simulink library "nort_sysgenlib"  (Simulink 6.5)
undefined symbols (not defined in the file or in its folder): Down, Up
libraries: xbsIndex_r4 x338, nort_sysgenlib x10
(part 2 of 2)

== system nort_sysgenlib/UnConcat32 ==
  note: Unconcat32: March 7, 2008
  In32 : Inport
  Convert : xbsIndex_r4/Convert  arith_type="Signed  (2's comp)"  n_bits=32  bin_pt=0  quantization=Truncate  overflow=Wrap  latency=0  dbl_ovrd=off  pipeline=off  block_type=convert
      settings: block_version=9.2.01
  Convert1 : xbsIndex_r4/Convert  arith_type="Signed  (2's comp)"  n_bits=32  bin_pt=0  quantization=Truncate  overflow=Wrap  latency=0  dbl_ovrd=off  pipeline=off  block_type=convert
      settings: block_version=9.2.01
  Convert2 : xbsIndex_r4/Convert  arith_type="Signed  (2's comp)"  n_bits=32  bin_pt=0  quantization=Truncate  overflow=Wrap  latency=0  dbl_ovrd=off  pipeline=off  block_type=convert
      settings: block_version=9.2.01
  Slice3 : xbsIndex_r4/Slice  nbits=32  boolean_output=off  mode=Lower Bit Location + Width  bit1=0  base1=MSB of Input  bit0=64  base0=LSB of Input  dbl_ovrd=off  block_type=slice
      settings: infoedit="Extracts a given range of bits from each input sample and presents it at the output.  The output type is ordinarily unsigned with binary point at zero, but can be Boolean when the slice is one bit wide.<P><P>Hardware notes: In hardware this block costs nothing."  block_version=9.2.01
  Slice4 : xbsIndex_r4/Slice  nbits=32  boolean_output=off  mode=Lower Bit Location + Width  bit1=0  base1=MSB of Input  bit0=32  base0=LSB of Input  dbl_ovrd=off  block_type=slice
      settings: infoedit="Extracts a given range of bits from each input sample and presents it at the output.  The output type is ordinarily unsigned with binary point at zero, but can be Boolean when the slice is one bit wide.<P><P>Hardware notes: In hardware this block costs nothing."  block_version=9.2.01
  Slice5 : xbsIndex_r4/Slice  nbits=32  boolean_output=off  mode=Lower Bit Location + Width  bit1=0  base1=MSB of Input  bit0=0  base0=LSB of Input  dbl_ovrd=off  block_type=slice
      settings: infoedit="Extracts a given range of bits from each input sample and presents it at the output.  The output type is ordinarily unsigned with binary point at zero, but can be Boolean when the slice is one bit wide.<P><P>Hardware notes: In hardware this block costs nothing."  block_version=9.2.01
  Out0 : Outport
  Out1 : Outport  Port=2
  Out2 : Outport  Port=3
  wires:
  Convert2/1 -> Out2/1
  Convert1/1 -> Out1/1
  Convert/1 -> Out0/1
  Slice5/1 -> Convert2/1
  Slice4/1 -> Convert1/1
  Slice3/1 -> Convert/1
  In32/1 -> Slice5/1, Slice4/1, Slice3/1

== system nort_sysgenlib/arp_ssp ==
  LVDS : Inport
  Signal : Outport
  ADOOR : Outport  Port=2
  wires:
  LVDS/1 -> Signal/1

== system nort_sysgenlib/ssp_ad_preaddr ==
  Signal : Inport
  ADOOR : Inport  Port=2
  TrigLevel : Inport  Port=3
  NAvg : Inport  Port=4
  RE : Inport  Port=5
  Reset : Inport  Port=6
  Trigger : Inport  Port=7
  PA_Out : Outport
  LvlGreater : Outport  Port=2
  wires:
  Signal/1 -> PA_Out/1

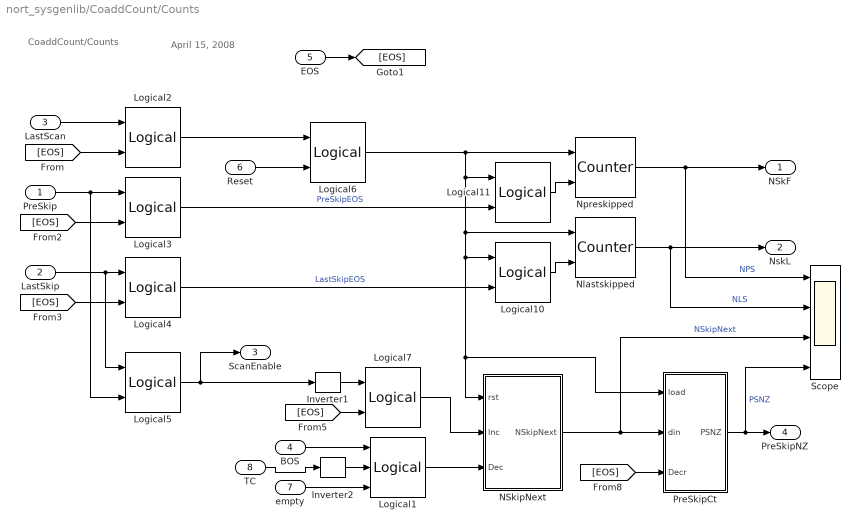
== system nort_sysgenlib/CoaddCount/Counts ==
  note: April 15, 2008
  note: CoaddCount/Counts
  PreSkip : Inport
  LastSkip : Inport  Port=2
  LastScan : Inport  Port=3
  BOS : Inport  Port=4
  EOS : Inport  Port=5
  Reset : Inport  Port=6
  empty : Inport  Port=7
  TC : Inport  Port=8
  Inverter1 : xbsIndex_r4/Inverter  en=off  latency=0  dbl_ovrd=off  block_type=inv
      settings: block_version=9.2.01
  Inverter2 : xbsIndex_r4/Inverter  en=off  latency=0  dbl_ovrd=off  block_type=inv
      settings: block_version=9.2.01
  Logical1 : xbsIndex_r4/Logical  logical_function=AND  inputs=3  en=off  latency=0  precision=Full  arith_type=Unsigned  n_bits=16  bin_pt=0  align_bp=on  dbl_ovrd=off  block_type=logical
      settings: block_version=9.2.01
  Logical10 : xbsIndex_r4/Logical  logical_function=OR  inputs=2  en=off  latency=0  precision=Full  arith_type=Unsigned  n_bits=16  bin_pt=0  align_bp=on  dbl_ovrd=off  block_type=logical
      settings: block_version=9.2.01
  Logical11 : xbsIndex_r4/Logical  logical_function=OR  inputs=2  en=off  latency=0  precision=Full  arith_type=Unsigned  n_bits=16  bin_pt=0  align_bp=on  dbl_ovrd=off  block_type=logical
      settings: block_version=9.2.01
  Logical{2..4,7} (4 alike) : xbsIndex_r4/Logical  logical_function=AND  inputs=2  en=off  latency=0  precision=Full  arith_type=Unsigned  n_bits=16  bin_pt=0  align_bp=on  dbl_ovrd=off  block_type=logical
      settings: block_version=9.2.01
  Logical5 : xbsIndex_r4/Logical  logical_function=NOR  inputs=2  en=off  latency=0  precision=Full  arith_type=Unsigned  n_bits=16  bin_pt=0  align_bp=on  dbl_ovrd=off  block_type=logical
      settings: block_version=9.2.01
  Logical6 : xbsIndex_r4/Logical  logical_function=OR  inputs=2  en=off  latency=0  precision=Full  arith_type=Unsigned  n_bits=16  bin_pt=0  align_bp=on  dbl_ovrd=off  block_type=logical
      settings: block_version=9.2.01
  NSkipNext : Subsystem
  Nlastskipped : xbsIndex_r4/Counter  cnt_type=Free Running  cnt_to=Inf  operation=Up  start_count=0  cnt_by_val=1  arith_type=Unsigned  n_bits=16  bin_pt=0  load_pin=off  rst=on  en=on  explicit_period=on  period=1  dbl_ovrd=off  use_behavioral_HDL=off  use_rpm=off  block_type=counter
      settings: block_version=9.2.01
  Npreskipped : xbsIndex_r4/Counter  cnt_type=Free Running  cnt_to=Inf  operation=Up  start_count=0  cnt_by_val=1  arith_type=Unsigned  n_bits=16  bin_pt=0  load_pin=off  rst=on  en=on  explicit_period=on  period=1  dbl_ovrd=off  use_behavioral_HDL=off  use_rpm=off  block_type=counter
      settings: block_version=9.2.01
  PreSkipCt : Subsystem
  Scope : Scope  NumInputPorts=4
      settings: TimeRange=5000  YMin=-0.25~-5~0~-5  YMax=1.25~5~15~5
  NSkF : Outport
  NskL : Outport  Port=2
  ScanEnable : Outport  Port=3
  PreSkipNZ : Outport  Port=4
  wires:
  Logical1/1 -> NSkipNext/3(Dec)
  empty/1 -> Logical1/3
  TC/1 -> Inverter2/1
  Inverter2/1 -> Logical1/2
  BOS/1 -> Logical1/1
  Logical7/1 -> NSkipNext/2(Inc)
  [EOS] -> Logical7/2
  Inverter1/1 -> Logical7/1
  [EOS] -> PreSkipCt/3(Decr)
  Reset/1 -> Logical6/2
  [EOS] -> Logical4/2
  [EOS] -> Logical3/2
  LastScan/1 -> Logical2/1
  [EOS] -> Logical2/2
  Logical6/1 -> Npreskipped/1, Nlastskipped/1, NSkipNext/1(rst), PreSkipCt/1(load), Logical10/1, Logical11/1
  Logical2/1 -> Logical6/1
  LastSkip/1 -> Logical5/1, Logical4/1
  Logical4/1 -> Logical10/2  "LastSkipEOS"
  Logical3/1 -> Logical11/2  "PreSkipEOS"
  PreSkip/1 -> Logical5/2, Logical3/1
  Logical5/1 -> Inverter1/1, ScanEnable/1
  PreSkipCt/1(PSNZ) -> Scope/4, PreSkipNZ/1  "PSNZ"
  EOS/1 -> [EOS]
  NSkipNext/1(NSkipNext) -> Scope/3, PreSkipCt/2(din)  "NSkipNext"
  Nlastskipped/1 -> Scope/2, NskL/1  "NLS"
  Npreskipped/1 -> Scope/1, NSkF/1  "NPS"
  Logical10/1 -> Nlastskipped/2
  Logical11/1 -> Npreskipped/2

== system nort_sysgenlib/CoaddCount/ScanCount ==
  note: March 6, 2008
  note: CoaddCount/ScanCount
  rst : Inport
  NC : Inport  Port=2
  en : Inport  Port=3
  Ncoadding : xbsIndex_r4/Counter  cnt_type=Free Running  cnt_to=Inf  operation=Up  start_count=1  cnt_by_val=1  arith_type=Unsigned  n_bits=14  bin_pt=0  load_pin=off  rst=on  en=on  explicit_period=on  period=1  dbl_ovrd=off  use_behavioral_HDL=off  use_rpm=off  block_type=counter
      settings: block_version=9.2.01
  Relational : xbsIndex_r4/Relational  mode=a=b  en=off  latency=0  dbl_ovrd=off  block_type=relational
      settings: block_version=9.2.01
  TC : Outport
  wires:
  en/1 -> Ncoadding/2
  Relational/1 -> TC/1
  rst/1 -> Ncoadding/1
  Ncoadding/1 -> Relational/2
  NC/1 -> Relational/1

== system nort_sysgenlib/PreAdder/Count ==
  note: February 27, 2008
  note: ssp_ad_preaddr/State
      | Simplified 2/27
      | EOSum is true on TC only
  NA : Inport
  Reset : Inport  Port=2
  Constant : xbsIndex_r4/Constant  arith_type=Unsigned  const=0  n_bits=7  bin_pt=0  explicit_period=off  period=1  equ=P=C  opselect=C  inp2=PCIN>>17  opr=+  inp1=P  carry=CIN  dbl_ovrd=off  block_type=constant
      settings: block_version=9.1.01
  Counter : xbsIndex_r4/Counter  cnt_type=Free Running  cnt_to=Inf  operation=Down  start_count=0  cnt_by_val=1  arith_type=Unsigned  n_bits=8  bin_pt=0  load_pin=on  rst=off  en=off  explicit_period=on  period=1  dbl_ovrd=off  use_behavioral_HDL=off  use_rpm=off  block_type=counter
      settings: block_version=9.1.01
  Inverter : xbsIndex_r4/Inverter  en=off  latency=0  dbl_ovrd=off  block_type=inv
      settings: block_version=9.2.01
  Logical : xbsIndex_r4/Logical  logical_function=OR  inputs=2  en=off  latency=0  precision=Full  arith_type=Unsigned  n_bits=16  bin_pt=0  align_bp=on  dbl_ovrd=off  block_type=logical
      settings: block_version=9.2.01
  Logical1 : xbsIndex_r4/Logical  logical_function=AND  inputs=2  en=off  latency=0  precision=Full  arith_type=Unsigned  n_bits=16  bin_pt=0  align_bp=on  dbl_ovrd=off  block_type=logical
      settings: block_version=9.2.01
  Relational : xbsIndex_r4/Relational  mode=a=b  en=off  latency=0  dbl_ovrd=off  block_type=relational
      settings: block_version=9.1.01
  NewData : Outport
  wires:
  Inverter/1 -> Logical1/2
  Logical1/1 -> NewData/1
  Logical/1 -> Counter/1
  Reset/1 -> Inverter/1, Logical/2  "Reset"
  NA/1 -> Counter/2
  Relational/1 -> Logical1/1, Logical/1  "TC"
  Constant/1 -> Relational/2
  Counter/1 -> Relational/1

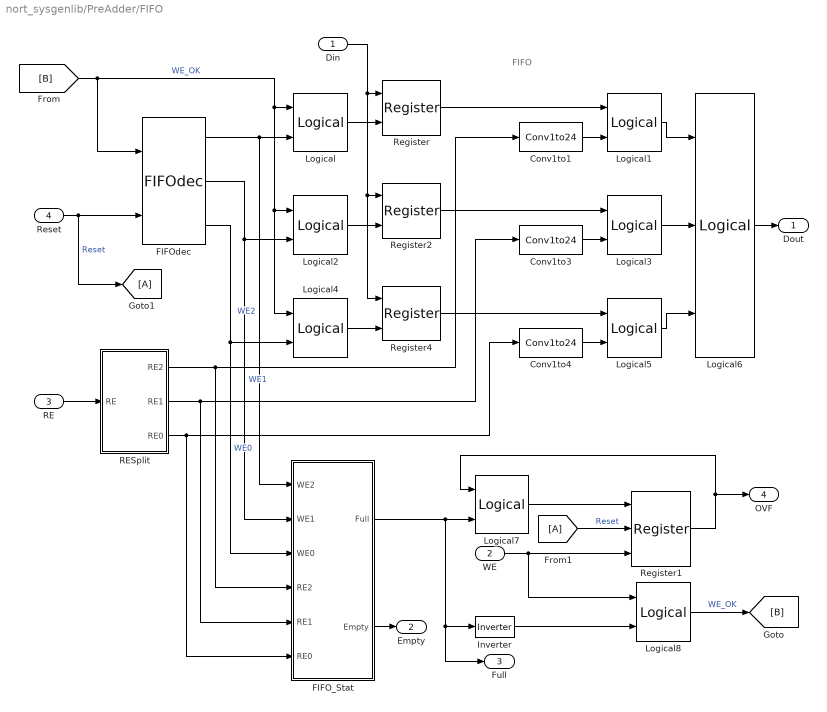
== system nort_sysgenlib/PreAdder/FIFO ==
  note: FIFO
  Din : Inport
  WE : Inport  Port=2
  RE : Inport  Port=3
  Reset : Inport  Port=4
  Conv1to1 : nort_sysgenlib/Conv1to24  SystemSampleTime=-1
  Conv1to3 : nort_sysgenlib/Conv1to24  SystemSampleTime=-1
  Conv1to4 : nort_sysgenlib/Conv1to24  SystemSampleTime=-1
  FIFO_Stat : Subsystem
  FIFOdec : nort_sysgenlib/FIFOdec  SystemSampleTime=-1
  Inverter : xbsIndex_r4/Inverter  en=off  latency=0  dbl_ovrd=off  block_type=inv
      settings: block_version=9.2.01
  Logical{,1..5,8} (7 alike) : xbsIndex_r4/Logical  logical_function=AND  inputs=2  en=off  latency=0  precision=Full  arith_type=Unsigned  n_bits=16  bin_pt=0  align_bp=on  dbl_ovrd=off  block_type=logical
      settings: block_version=9.2.01
  Logical6 : xbsIndex_r4/Logical  logical_function=OR  inputs=3  en=off  latency=0  precision=Full  arith_type=Unsigned  n_bits=16  bin_pt=0  align_bp=on  dbl_ovrd=off  block_type=logical
      settings: block_version=9.2.01
  Logical7 : xbsIndex_r4/Logical  logical_function=OR  inputs=2  en=off  latency=0  precision=Full  arith_type=Unsigned  n_bits=16  bin_pt=0  align_bp=on  dbl_ovrd=off  block_type=logical
      settings: block_version=9.2.01
  RESplit : Subsystem
  Register : xbsIndex_r4/Register  init=0  rst=off  en=on  dbl_ovrd=off  block_type=register
      settings: block_version=9.2.01
  Register1 : xbsIndex_r4/Register  init=0  rst=on  en=on  dbl_ovrd=off  block_type=register
      settings: block_version=9.2.01
  Register2 : xbsIndex_r4/Register  init=0  rst=off  en=on  dbl_ovrd=off  block_type=register
      settings: block_version=9.2.01
  Register4 : xbsIndex_r4/Register  init=0  rst=off  en=on  dbl_ovrd=off  block_type=register
      settings: block_version=9.2.01
  Dout : Outport
  Empty : Outport  Port=2
  Full : Outport  Port=3
  OVF : Outport  Port=4
  wires:
  [B] -> FIFOdec/1, Logical2/1, Logical4/1, Logical/1  "WE_OK"
  Logical8/1 -> [B]  "WE_OK"
  [A] -> Register1/2  "Reset"
  Inverter/1 -> Logical8/2
  FIFO_Stat/1(Full) -> Full/1, Inverter/1, Logical7/2
  FIFO_Stat/2(Empty) -> Empty/1
  Logical7/1 -> Register1/1
  WE/1 -> Logical8/1, Register1/3
  Register1/1 -> Logical7/1, OVF/1
  RE/1 -> RESplit/1(RE)
  Reset/1 -> FIFOdec/2, [A]  "Reset"
  Logical6/1 -> Dout/1
  Logical5/1 -> Logical6/3
  Logical3/1 -> Logical6/2
  Logical1/1 -> Logical6/1
  RESplit/1(RE2) -> FIFO_Stat/4(RE2), Conv1to1/1
  Register4/1 -> Logical5/1
  Register2/1 -> Logical3/1
  Conv1to4/1 -> Logical5/2
  FIFOdec/3 -> FIFO_Stat/3(WE0), Logical4/2  "WE0"
  Logical4/1 -> Register4/2
  Conv1to3/1 -> Logical3/2
  FIFOdec/2 -> FIFO_Stat/2(WE1), Logical2/2  "WE1"
  Logical2/1 -> Register2/2
  Register/1 -> Logical1/1
  Conv1to1/1 -> Logical1/2
  RESplit/3(RE0) -> FIFO_Stat/6(RE0), Conv1to4/1
  RESplit/2(RE1) -> FIFO_Stat/5(RE1), Conv1to3/1
  FIFOdec/1 -> FIFO_Stat/1(WE2), Logical/2  "WE2"
  Din/1 -> Register4/1, Register2/1, Register/1
  Logical/1 -> Register/2

== system nort_sysgenlib/PreAdder/State ==
  note: February 27, 2008
  note: PreAdder State
  ResIn : Inport
  Trigger : Inport  Port=2
  ActiveSt : xbsIndex_r4/Register  init=0  rst=off  en=off  dbl_ovrd=off  block_type=register
      settings: block_version=9.2.01
  Armed : xbsIndex_r4/Register  init=0  rst=off  en=off  dbl_ovrd=off  block_type=register
      settings: block_version=9.2.01
  Inverter1 : xbsIndex_r4/Inverter  en=off  latency=0  dbl_ovrd=off  block_type=inv
      settings: block_version=9.2.01
  Inverter2 : xbsIndex_r4/Inverter  en=off  latency=0  dbl_ovrd=off  block_type=inv
      settings: block_version=9.2.01
  Inverter3 : xbsIndex_r4/Inverter  en=off  latency=0  dbl_ovrd=off  block_type=inv
      settings: block_version=9.2.01
  Logical{1,4,6..7} (4 alike) : xbsIndex_r4/Logical  logical_function=AND  inputs=2  en=off  latency=0  precision=Full  arith_type=Unsigned  n_bits=16  bin_pt=0  align_bp=on  dbl_ovrd=off  block_type=logical
      settings: block_version=9.2.01
  Logical5 : xbsIndex_r4/Logical  logical_function=OR  inputs=2  en=off  latency=0  precision=Full  arith_type=Unsigned  n_bits=16  bin_pt=0  align_bp=on  dbl_ovrd=off  block_type=logical
      settings: block_version=9.2.01
  Logical8 : xbsIndex_r4/Logical  logical_function=OR  inputs=2  en=off  latency=0  precision=Full  arith_type=Unsigned  n_bits=16  bin_pt=0  align_bp=on  dbl_ovrd=off  block_type=logical
      settings: block_version=9.2.01
  ResetSt : xbsIndex_r4/Register  init=0  rst=off  en=off  dbl_ovrd=off  block_type=register
      settings: block_version=9.2.01
  Inactive : Outport
  Reset : Outport  Port=2
  wires:
  Inverter2/1 -> Inactive/1
  Logical1/1 -> Logical8/1
  Inverter3/1 -> Logical6/1
  Logical8/1 -> Logical7/2
  Logical7/1 -> Inverter2/1, ActiveSt/1
  ActiveSt/1 -> Logical8/2
  Armed/1 -> Logical1/1, Logical6/2
  Logical6/1 -> Logical5/2
  Logical5/1 -> Logical4/1
  Inverter1/1 -> Logical4/2, Logical7/1
  Logical4/1 -> Armed/1
  ResIn/1 -> ResetSt/1, Inverter1/1  "Reset_In"
  Trigger/1 -> Logical1/2, Inverter3/1  "Trigger"
  ResetSt/1 -> Logical5/1, Reset/1

== system nort_sysgenlib/PreAdderA/Count ==
  note: April 16, 2008
  note: ssp_ad_preaddr/State
      | Simplified 2/27
      | EOSum is true on TC only
  Reset : Inport
  NA : Inport  Port=2
  Constant : xbsIndex_r4/Constant  arith_type=Unsigned  const=0  n_bits=7  bin_pt=0  explicit_period=off  period=1  equ=P=C  opselect=C  inp2=PCIN>>17  opr=+  inp1=P  carry=CIN  dbl_ovrd=off  block_type=constant
      settings: block_version=9.1.01
  Counter : xbsIndex_r4/Counter  cnt_type=Free Running  cnt_to=Inf  operation=Down  start_count=0  cnt_by_val=1  arith_type=Unsigned  n_bits=8  bin_pt=0  load_pin=on  rst=off  en=off  explicit_period=on  period=1  dbl_ovrd=off  use_behavioral_HDL=off  use_rpm=off  block_type=counter
      settings: block_version=9.1.01
  Inverter : xbsIndex_r4/Inverter  en=off  latency=0  dbl_ovrd=off  block_type=inv
      settings: block_version=9.2.01
  Logical : xbsIndex_r4/Logical  logical_function=OR  inputs=2  en=off  latency=0  precision=Full  arith_type=Unsigned  n_bits=16  bin_pt=0  align_bp=on  dbl_ovrd=off  block_type=logical
      settings: block_version=9.2.01
  Logical1 : xbsIndex_r4/Logical  logical_function=AND  inputs=2  en=off  latency=0  precision=Full  arith_type=Unsigned  n_bits=16  bin_pt=0  align_bp=on  dbl_ovrd=off  block_type=logical
      settings: block_version=9.2.01
  Relational : xbsIndex_r4/Relational  mode=a=b  en=off  latency=0  dbl_ovrd=off  block_type=relational
      settings: block_version=9.1.01
  NewData : Outport
  wires:
  Inverter/1 -> Logical1/2
  Logical1/1 -> NewData/1
  Logical/1 -> Counter/1
  Reset/1 -> Inverter/1, Logical/2  "Reset"
  NA/1 -> Counter/2
  Relational/1 -> Logical1/1, Logical/1  "TC"
  Constant/1 -> Relational/2
  Counter/1 -> Relational/1

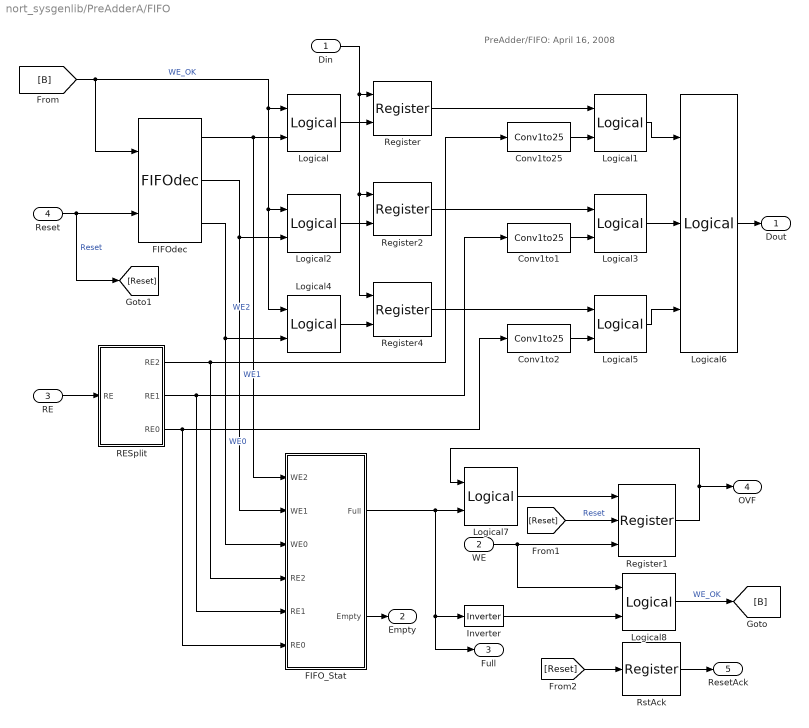
== system nort_sysgenlib/PreAdderA/FIFO ==
  note: PreAdder/FIFO: April 16, 2008
  Din : Inport
  WE : Inport  Port=2
  RE : Inport  Port=3
  Reset : Inport  Port=4
  Conv1to1 : nort_sysgenlib/Conv1to25  SystemSampleTime=-1
  Conv1to2 : nort_sysgenlib/Conv1to25  SystemSampleTime=-1
  Conv1to25 : nort_sysgenlib/Conv1to25  SystemSampleTime=-1
  FIFO_Stat : Subsystem
  FIFOdec : nort_sysgenlib/FIFOdec  SystemSampleTime=-1
  Inverter : xbsIndex_r4/Inverter  en=off  latency=0  dbl_ovrd=off  block_type=inv
      settings: block_version=9.2.01
  Logical{,1..5,8} (7 alike) : xbsIndex_r4/Logical  logical_function=AND  inputs=2  en=off  latency=0  precision=Full  arith_type=Unsigned  n_bits=16  bin_pt=0  align_bp=on  dbl_ovrd=off  block_type=logical
      settings: block_version=9.2.01
  Logical6 : xbsIndex_r4/Logical  logical_function=OR  inputs=3  en=off  latency=0  precision=Full  arith_type=Unsigned  n_bits=16  bin_pt=0  align_bp=on  dbl_ovrd=off  block_type=logical
      settings: block_version=9.2.01
  Logical7 : xbsIndex_r4/Logical  logical_function=OR  inputs=2  en=off  latency=0  precision=Full  arith_type=Unsigned  n_bits=16  bin_pt=0  align_bp=on  dbl_ovrd=off  block_type=logical
      settings: block_version=9.2.01
  RESplit : Subsystem
  Register : xbsIndex_r4/Register  init=0  rst=off  en=on  dbl_ovrd=off  block_type=register
      settings: block_version=9.2.01
  Register1 : xbsIndex_r4/Register  init=0  rst=on  en=on  dbl_ovrd=off  block_type=register
      settings: block_version=9.2.01
  Register2 : xbsIndex_r4/Register  init=0  rst=off  en=on  dbl_ovrd=off  block_type=register
      settings: block_version=9.2.01
  Register4 : xbsIndex_r4/Register  init=0  rst=off  en=on  dbl_ovrd=off  block_type=register
      settings: block_version=9.2.01
  RstAck : xbsIndex_r4/Register  init=0  rst=off  en=off  dbl_ovrd=off  block_type=register
      settings: block_version=9.2.01
  Dout : Outport
  Empty : Outport  Port=2
  Full : Outport  Port=3
  OVF : Outport  Port=4
  ResetAck : Outport  Port=5
  wires:
  [Reset] -> RstAck/1
  RstAck/1 -> ResetAck/1
  [B] -> FIFOdec/1, Logical2/1, Logical4/1, Logical/1  "WE_OK"
  Logical8/1 -> [B]  "WE_OK"
  [Reset] -> Register1/2  "Reset"
  Inverter/1 -> Logical8/2
  FIFO_Stat/1(Full) -> Full/1, Inverter/1, Logical7/2
  FIFO_Stat/2(Empty) -> Empty/1
  Logical7/1 -> Register1/1
  WE/1 -> Logical8/1, Register1/3
  Register1/1 -> Logical7/1, OVF/1
  RE/1 -> RESplit/1(RE)
  Reset/1 -> FIFOdec/2, [Reset]  "Reset"
  Logical6/1 -> Dout/1
  Logical5/1 -> Logical6/3
  Logical3/1 -> Logical6/2
  Logical1/1 -> Logical6/1
  RESplit/1(RE2) -> FIFO_Stat/4(RE2), Conv1to25/1
  Register4/1 -> Logical5/1
  Register2/1 -> Logical3/1
  Conv1to2/1 -> Logical5/2
  FIFOdec/3 -> FIFO_Stat/3(WE0), Logical4/2  "WE0"
  Logical4/1 -> Register4/2
  Conv1to1/1 -> Logical3/2
  FIFOdec/2 -> FIFO_Stat/2(WE1), Logical2/2  "WE1"
  Logical2/1 -> Register2/2
  Register/1 -> Logical1/1
  Conv1to25/1 -> Logical1/2
  RESplit/3(RE0) -> FIFO_Stat/6(RE0), Conv1to2/1
  RESplit/2(RE1) -> FIFO_Stat/5(RE1), Conv1to1/1
  FIFOdec/1 -> FIFO_Stat/1(WE2), Logical/2  "WE2"
  Din/1 -> Register4/1, Register2/1, Register/1
  Logical/1 -> Register/2

== system nort_sysgenlib/PreAdderA/State ==
  note: April 16, 2008
  note: PreAdder State
  Trigger : Inport
  ResIn : Inport  Port=2
  ActiveSt : xbsIndex_r4/Register  init=0  rst=off  en=off  dbl_ovrd=off  block_type=register
      settings: block_version=9.2.01
  Armed : xbsIndex_r4/Register  init=0  rst=off  en=off  dbl_ovrd=off  block_type=register
      settings: block_version=9.2.01
  Inverter1 : xbsIndex_r4/Inverter  en=off  latency=0  dbl_ovrd=off  block_type=inv
      settings: block_version=9.2.01
  Inverter2 : xbsIndex_r4/Inverter  en=off  latency=0  dbl_ovrd=off  block_type=inv
      settings: block_version=9.2.01
  Inverter3 : xbsIndex_r4/Inverter  en=off  latency=0  dbl_ovrd=off  block_type=inv
      settings: block_version=9.2.01
  Logical{1,4,6..7} (4 alike) : xbsIndex_r4/Logical  logical_function=AND  inputs=2  en=off  latency=0  precision=Full  arith_type=Unsigned  n_bits=16  bin_pt=0  align_bp=on  dbl_ovrd=off  block_type=logical
      settings: block_version=9.2.01
  Logical5 : xbsIndex_r4/Logical  logical_function=OR  inputs=2  en=off  latency=0  precision=Full  arith_type=Unsigned  n_bits=16  bin_pt=0  align_bp=on  dbl_ovrd=off  block_type=logical
      settings: block_version=9.2.01
  Logical8 : xbsIndex_r4/Logical  logical_function=OR  inputs=2  en=off  latency=0  precision=Full  arith_type=Unsigned  n_bits=16  bin_pt=0  align_bp=on  dbl_ovrd=off  block_type=logical
      settings: block_version=9.2.01
  ResetSt : xbsIndex_r4/Register  init=0  rst=off  en=off  dbl_ovrd=off  block_type=register
      settings: block_version=9.2.01
  Inactive : Outport
  Reset : Outport  Port=2
  wires:
  Inverter2/1 -> Inactive/1
  Logical1/1 -> Logical8/1
  Inverter3/1 -> Logical6/1
  Logical8/1 -> Logical7/2
  Logical7/1 -> Inverter2/1, ActiveSt/1
  ActiveSt/1 -> Logical8/2
  Armed/1 -> Logical1/1, Logical6/2
  Logical6/1 -> Logical5/2
  Logical5/1 -> Logical4/1
  Inverter1/1 -> Logical4/2, Logical7/1
  Logical4/1 -> Armed/1
  ResIn/1 -> ResetSt/1, Inverter1/1  "Reset_In"
  Trigger/1 -> Logical1/2, Inverter3/1  "Trigger"
  ResetSt/1 -> Logical5/1, Reset/1

== system nort_sysgenlib/StateShifter/MuxAddrCalc ==
  note: MuxAddrCalc: March 7, 2008
  SHsel : Inport
  St0 : Inport  Port=2
  St1 : Inport  Port=3
  St2 : Inport  Port=4
  AddSub : xbsIndex_r4/AddSub  mode=Addition  use_carryin=off  use_carryout=off  en=off  latency=0  precision=Full  arith_type=Unsigned  n_bits=16  bin_pt=14  quantization=Truncate  overflow=Wrap  dbl_ovrd=off  use_behavioral_HDL=off  pipelined=off  use_rpm=on  block_type=addsub
      settings: block_version=9.2.01
  Concat : xbsIndex_r4/Concat  num_inputs=2  dbl_ovrd=off  block_type=concat
      settings: block_version=9.2.01
  Logical1 : xbsIndex_r4/Logical  logical_function=OR  inputs=2  en=off  latency=0  precision=Full  arith_type=Unsigned  n_bits=16  bin_pt=0  align_bp=on  dbl_ovrd=off  block_type=logical
      settings: block_version=9.2.01
  Logical2 : xbsIndex_r4/Logical  logical_function=OR  inputs=2  en=off  latency=0  precision=Full  arith_type=Unsigned  n_bits=16  bin_pt=0  align_bp=on  dbl_ovrd=off  block_type=logical
      settings: block_version=9.2.01
  MuxSel : Outport
  wires:
  St0/1 -> Logical1/1
  St1/1 -> Logical2/1
  AddSub/1 -> MuxSel/1
  SHsel/1 -> AddSub/1
  Concat/1 -> AddSub/2
  Logical1/1 -> Concat/2
  Logical2/1 -> Concat/1
  St2/1 -> Logical2/2, Logical1/2

== system nort_sysgenlib/StateShifter/ShiftHeader ==
  note: March 7, 2008
  note: ShiftHeader
  StI : Inport
  StSH : Inport  Port=2
  notfull : Inport  Port=3
  Constant : xbsIndex_r4/Constant  arith_type=Unsigned  const=5  n_bits=4  bin_pt=0  explicit_period=off  period=1  equ=P=C  opselect=C  inp2=PCIN>>17  opr=+  inp1=P  carry=CIN  dbl_ovrd=off  block_type=constant
      settings: block_version=9.2.01
  Counter : xbsIndex_r4/Counter  cnt_type=Free Running  cnt_to=Inf  operation=Up  start_count=0  cnt_by_val=1  arith_type=Unsigned  n_bits=3  bin_pt=0  load_pin=off  rst=on  en=on  explicit_period=on  period=1  dbl_ovrd=off  use_behavioral_HDL=off  use_rpm=off  block_type=counter
      settings: block_version=9.2.01
  Logical1 : xbsIndex_r4/Logical  logical_function=AND  inputs=2  en=off  latency=0  precision=Full  arith_type=Unsigned  n_bits=16  bin_pt=0  align_bp=on  dbl_ovrd=off  block_type=logical
      settings: block_version=9.2.01
  Logical2 : xbsIndex_r4/Logical  logical_function=AND  inputs=2  en=off  latency=0  precision=Full  arith_type=Unsigned  n_bits=16  bin_pt=0  align_bp=on  dbl_ovrd=off  block_type=logical
      settings: block_version=9.2.01
  Relational : xbsIndex_r4/Relational  mode=a=b  en=off  latency=0  dbl_ovrd=off  block_type=relational
      settings: block_version=9.2.01
  SHdone : Outport
  SHSel : Outport  Port=2
  wires:
  Logical2/1 -> SHdone/1
  Relational/1 -> Logical2/1
  Constant/1 -> Relational/2
  notfull/1 -> Logical2/2, Logical1/2
  StSH/1 -> Logical1/1
  StI/1 -> Counter/1
  Logical1/1 -> Counter/2
  Counter/1 -> SHSel/1, Relational/1

== system nort_sysgenlib/Triggering/AutoTrig ==
  note: AutoTrigger Circuit: May 28, 2008
  Trig : Inport
  AutoEn : Inport  Port=2
  Constant : xbsIndex_r4/Constant  arith_type=Unsigned  const=0  n_bits=9  bin_pt=0  explicit_period=off  period=1  equ=P=C  opselect=C  inp2=PCIN>>17  opr=+  inp1=P  carry=CIN  dbl_ovrd=off  block_type=constant
      settings: block_version=9.1.01
  Counter : xbsIndex_r4/Counter  cnt_type=Free Running  cnt_to=Inf  operation=Down  start_count=10000000  cnt_by_val=1  arith_type=Unsigned  n_bits=24  bin_pt=0  load_pin=off  rst=on  en=off  explicit_period=on  period=1  dbl_ovrd=off  use_behavioral_HDL=off  use_rpm=off  block_type=counter
      settings: block_version=9.1.01
  Delay : xbsIndex_r4/Delay  en=off  latency=1  dbl_ovrd=off  reg_retiming=off  block_type=delay
      settings: block_version=9.2.01
  Inverter : xbsIndex_r4/Inverter  en=off  latency=0  dbl_ovrd=off  block_type=inv
      settings: block_version=9.1.01
  Inverter1 : xbsIndex_r4/Inverter  en=off  latency=0  dbl_ovrd=off  block_type=inv
      settings: block_version=9.2.01
  Logical1 : xbsIndex_r4/Logical  logical_function=AND  inputs=2  en=off  latency=0  precision=Full  arith_type=Unsigned  n_bits=16  bin_pt=0  align_bp=on  dbl_ovrd=off  block_type=logical
      settings: block_version=9.1.01
  Logical2 : xbsIndex_r4/Logical  logical_function=OR  inputs=2  en=off  latency=0  precision=Full  arith_type=Unsigned  n_bits=16  bin_pt=0  align_bp=on  dbl_ovrd=off  block_type=logical
      settings: block_version=9.1.01
  Logical3 : xbsIndex_r4/Logical  logical_function=AND  inputs=2  en=off  latency=0  precision=Full  arith_type=Unsigned  n_bits=16  bin_pt=0  align_bp=on  dbl_ovrd=off  block_type=logical
      settings: block_version=9.1.01
  Logical4 : xbsIndex_r4/Logical  logical_function=AND  inputs=2  en=off  latency=0  precision=Full  arith_type=Unsigned  n_bits=16  bin_pt=0  align_bp=on  dbl_ovrd=off  block_type=logical
      settings: block_version=9.1.01
  Relational : xbsIndex_r4/Relational  mode=a=b  en=off  latency=0  dbl_ovrd=off  block_type=relational
      settings: block_version=9.1.01
  AutoTrig : Outport
  wires:
  Logical4/1 -> AutoTrig/1
  Delay/1 -> Logical4/2
  Logical1/1 -> Delay/1
  Inverter1/1 -> Logical1/1
  Logical3/1 -> Logical4/1, Inverter1/1
  Trig/1 -> Logical2/1
  AutoEn/1 -> Logical1/2, Logical3/2, Inverter/1
  Inverter/1 -> Logical2/2
  Logical2/1 -> Counter/1
  Relational/1 -> Logical3/1
  Counter/1 -> Relational/1
  Constant/1 -> Relational/2

== system nort_sysgenlib/CoaddCount/Counts/NSkipNext ==
  note: CoaddCount/Counts/NSkipNext: April 16, 2008
  rst : Inport
  Inc : Inport  Port=2
  Dec : Inport  Port=3
  Constant1 : xbsIndex_r4/Constant  arith_type=Unsigned  const=0  n_bits=12  bin_pt=0  explicit_period=off  period=1  equ=P=C  opselect=C  inp2=PCIN>>17  opr=+  inp1=P  carry=CIN  dbl_ovrd=off  block_type=constant
      settings: block_version=9.2.01
  Logical1 : xbsIndex_r4/Logical  logical_function=OR  inputs=3  en=off  latency=0  precision=Full  arith_type=Unsigned  n_bits=16  bin_pt=0  align_bp=on  dbl_ovrd=off  block_type=logical
      settings: block_version=9.2.01
  Logical2 : xbsIndex_r4/Logical  logical_function=AND  inputs=2  en=off  latency=0  precision=Full  arith_type=Unsigned  n_bits=16  bin_pt=0  align_bp=on  dbl_ovrd=off  block_type=logical
      settings: block_version=9.2.01
  Ntoskipnext : xbsIndex_r4/Counter  cnt_type=Free Running  cnt_to=Inf  operation=Up/Down  start_count=0  cnt_by_val=1  arith_type=Unsigned  n_bits=16  bin_pt=0  load_pin=off  rst=on  en=on  explicit_period=on  period=1  dbl_ovrd=off  use_behavioral_HDL=off  use_rpm=off  block_type=counter
      settings: block_version=9.2.01
  Relational1 : xbsIndex_r4/Relational  mode=a!=b  en=off  latency=0  dbl_ovrd=off  block_type=relational
      settings: block_version=9.2.01
  NSkipNext : Outport
  wires:
  Logical2/1 -> Logical1/3
  Inc/1 -> Logical1/2, Ntoskipnext/1
  Relational1/1 -> Logical2/2
  Dec/1 -> Logical2/1
  Constant1/1 -> Relational1/2
  Ntoskipnext/1 -> Relational1/1, NSkipNext/1
  rst/1 -> Logical1/1, Ntoskipnext/2
  Logical1/1 -> Ntoskipnext/3

== system nort_sysgenlib/CoaddCount/Counts/PreSkipCt ==
  note: April 16, 2008
  note: PreSkipCt
  load : Inport
  din : Inport  Port=2
  Decr : Inport  Port=3
  Constant : xbsIndex_r4/Constant  arith_type=Unsigned  const=0  n_bits=12  bin_pt=0  explicit_period=off  period=1  equ=P=C  opselect=C  inp2=PCIN>>17  opr=+  inp1=P  carry=CIN  dbl_ovrd=off  block_type=constant
      settings: block_version=9.2.01
  Logical12 : xbsIndex_r4/Logical  logical_function=OR  inputs=2  en=off  latency=0  precision=Full  arith_type=Unsigned  n_bits=16  bin_pt=0  align_bp=on  dbl_ovrd=off  block_type=logical
      settings: block_version=9.2.01
  Logical14 : xbsIndex_r4/Logical  logical_function=AND  inputs=2  en=off  latency=0  precision=Full  arith_type=Unsigned  n_bits=16  bin_pt=0  align_bp=on  dbl_ovrd=off  block_type=logical
      settings: block_version=9.2.01
  PreSkipCt : xbsIndex_r4/Counter  cnt_type=Free Running  cnt_to=Inf  operation=Down  start_count=0  cnt_by_val=1  arith_type=Unsigned  n_bits=16  bin_pt=0  load_pin=on  rst=off  en=on  explicit_period=on  period=1  dbl_ovrd=off  use_behavioral_HDL=off  use_rpm=off  block_type=counter
      settings: block_version=9.2.01
  Relational : xbsIndex_r4/Relational  mode=a!=b  en=off  latency=0  dbl_ovrd=off  block_type=relational
      settings: block_version=9.2.01
  PSNZ : Outport
  wires:
  Decr/1 -> Logical14/1
  Relational/1 -> Logical14/2, PSNZ/1  "PSNZ"
  din/1 -> PreSkipCt/2
  load/1 -> PreSkipCt/1, Logical12/1
  Logical14/1 -> Logical12/2
  Logical12/1 -> PreSkipCt/3
  Constant/1 -> Relational/2
  PreSkipCt/1 -> Relational/1

== system nort_sysgenlib/PreAdder/FIFO/FIFO_Stat ==
  WE2 : Inport
  WE1 : Inport  Port=2
  WE0 : Inport  Port=3
  RE2 : Inport  Port=4
  RE1 : Inport  Port=5
  RE0 : Inport  Port=6
  Logical{1..2,4..6,8} (6 alike) : xbsIndex_r4/Logical  logical_function=AND  inputs=2  en=off  latency=0  precision=Full  arith_type=Unsigned  n_bits=16  bin_pt=0  align_bp=on  dbl_ovrd=off  block_type=logical
      settings: block_version=9.2.01
  Logical3 : xbsIndex_r4/Logical  logical_function=OR  inputs=3  en=off  latency=0  precision=Full  arith_type=Unsigned  n_bits=16  bin_pt=0  align_bp=on  dbl_ovrd=off  block_type=logical
      settings: block_version=9.2.01
  Logical7 : xbsIndex_r4/Logical  logical_function=OR  inputs=3  en=off  latency=0  precision=Full  arith_type=Unsigned  n_bits=16  bin_pt=0  align_bp=on  dbl_ovrd=off  block_type=logical
      settings: block_version=9.2.01
  Full : Outport
  Empty : Outport  Port=2
  wires:
  Logical7/1 -> Full/1
  Logical6/1 -> Logical7/3
  Logical5/1 -> Logical7/2
  Logical8/1 -> Logical7/1
  Logical3/1 -> Empty/1
  Logical2/1 -> Logical3/3
  Logical1/1 -> Logical3/2
  Logical4/1 -> Logical3/1
  RE2/1 -> Logical5/2, Logical4/2
  RE0/1 -> Logical8/2, Logical2/2
  WE0/1 -> Logical6/1, Logical2/1
  RE1/1 -> Logical6/2, Logical1/2
  WE1/1 -> Logical5/1, Logical1/1
  WE2/1 -> Logical8/1, Logical4/1

== system nort_sysgenlib/PreAdder/FIFO/RESplit ==
  RE : Inport
  Slice : xbsIndex_r4/Slice  nbits=1  boolean_output=on  mode=Lower Bit Location + Width  bit1=0  base1=MSB of Input  bit0=2  base0=LSB of Input  dbl_ovrd=off  block_type=slice
      settings: infoedit="Extracts a given range of bits from each input sample and presents it at the output.  The output type is ordinarily unsigned with binary point at zero, but can be Boolean when the slice is one bit wide.<P><P>Hardware notes: In hardware this block costs nothing."  block_version=9.2.01
  Slice1 : xbsIndex_r4/Slice  nbits=1  boolean_output=on  mode=Lower Bit Location + Width  bit1=0  base1=MSB of Input  bit0=1  base0=LSB of Input  dbl_ovrd=off  block_type=slice
      settings: infoedit="Extracts a given range of bits from each input sample and presents it at the output.  The output type is ordinarily unsigned with binary point at zero, but can be Boolean when the slice is one bit wide.<P><P>Hardware notes: In hardware this block costs nothing."  block_version=9.2.01
  Slice2 : xbsIndex_r4/Slice  nbits=1  boolean_output=on  mode=Lower Bit Location + Width  bit1=0  base1=MSB of Input  bit0=0  base0=LSB of Input  dbl_ovrd=off  block_type=slice
      settings: infoedit="Extracts a given range of bits from each input sample and presents it at the output.  The output type is ordinarily unsigned with binary point at zero, but can be Boolean when the slice is one bit wide.<P><P>Hardware notes: In hardware this block costs nothing."  block_version=9.2.01
  RE2 : Outport
  RE1 : Outport  Port=2
  RE0 : Outport  Port=3
  wires:
  Slice2/1 -> RE0/1
  Slice1/1 -> RE1/1
  Slice/1 -> RE2/1
  RE/1 -> Slice2/1, Slice1/1, Slice/1

== system nort_sysgenlib/PreAdderA/FIFO/FIFO_Stat ==
  WE2 : Inport
  WE1 : Inport  Port=2
  WE0 : Inport  Port=3
  RE2 : Inport  Port=4
  RE1 : Inport  Port=5
  RE0 : Inport  Port=6
  Logical{1..2,4..6,8} (6 alike) : xbsIndex_r4/Logical  logical_function=AND  inputs=2  en=off  latency=0  precision=Full  arith_type=Unsigned  n_bits=16  bin_pt=0  align_bp=on  dbl_ovrd=off  block_type=logical
      settings: block_version=9.2.01
  Logical3 : xbsIndex_r4/Logical  logical_function=OR  inputs=3  en=off  latency=0  precision=Full  arith_type=Unsigned  n_bits=16  bin_pt=0  align_bp=on  dbl_ovrd=off  block_type=logical
      settings: block_version=9.2.01
  Logical7 : xbsIndex_r4/Logical  logical_function=OR  inputs=3  en=off  latency=0  precision=Full  arith_type=Unsigned  n_bits=16  bin_pt=0  align_bp=on  dbl_ovrd=off  block_type=logical
      settings: block_version=9.2.01
  Full : Outport
  Empty : Outport  Port=2
  wires:
  Logical7/1 -> Full/1
  Logical6/1 -> Logical7/3
  Logical5/1 -> Logical7/2
  Logical8/1 -> Logical7/1
  Logical3/1 -> Empty/1
  Logical2/1 -> Logical3/3
  Logical1/1 -> Logical3/2
  Logical4/1 -> Logical3/1
  RE2/1 -> Logical5/2, Logical4/2
  RE0/1 -> Logical8/2, Logical2/2
  WE0/1 -> Logical6/1, Logical2/1
  RE1/1 -> Logical6/2, Logical1/2
  WE1/1 -> Logical5/1, Logical1/1
  WE2/1 -> Logical8/1, Logical4/1

== system nort_sysgenlib/PreAdderA/FIFO/RESplit ==
  RE : Inport
  Slice : xbsIndex_r4/Slice  nbits=1  boolean_output=on  mode=Lower Bit Location + Width  bit1=0  base1=MSB of Input  bit0=2  base0=LSB of Input  dbl_ovrd=off  block_type=slice
      settings: infoedit="Extracts a given range of bits from each input sample and presents it at the output.  The output type is ordinarily unsigned with binary point at zero, but can be Boolean when the slice is one bit wide.<P><P>Hardware notes: In hardware this block costs nothing."  block_version=9.2.01
  Slice1 : xbsIndex_r4/Slice  nbits=1  boolean_output=on  mode=Lower Bit Location + Width  bit1=0  base1=MSB of Input  bit0=1  base0=LSB of Input  dbl_ovrd=off  block_type=slice
      settings: infoedit="Extracts a given range of bits from each input sample and presents it at the output.  The output type is ordinarily unsigned with binary point at zero, but can be Boolean when the slice is one bit wide.<P><P>Hardware notes: In hardware this block costs nothing."  block_version=9.2.01
  Slice2 : xbsIndex_r4/Slice  nbits=1  boolean_output=on  mode=Lower Bit Location + Width  bit1=0  base1=MSB of Input  bit0=0  base0=LSB of Input  dbl_ovrd=off  block_type=slice
      settings: infoedit="Extracts a given range of bits from each input sample and presents it at the output.  The output type is ordinarily unsigned with binary point at zero, but can be Boolean when the slice is one bit wide.<P><P>Hardware notes: In hardware this block costs nothing."  block_version=9.2.01
  RE2 : Outport
  RE1 : Outport  Port=2
  RE0 : Outport  Port=3
  wires:
  Slice2/1 -> RE0/1
  Slice1/1 -> RE1/1
  Slice/1 -> RE2/1
  RE/1 -> Slice2/1, Slice1/1, Slice/1
